simulink model "chydrbf_bruite_s"  (R2025a)
settings: Solver=ode45  StartTime=0.0  StopTime=50  MaxStep=1  MinStep=0.0001  RelTol=1e-8  AbsTol=1e-8  EnableMultiTasking=on
values from neighbouring files (symbols this model uses):
  F = [1 7.33333333333 21.7708333333 37 33.0208333333 11.4583333333]    [datahydr.mat]    (also in part4.m = ppfil(B,Aa,Tf); ppfil.m = real(poly(diag(r))))
  kw = 0.5    [datahydr.mat]    (also in initchydr.m)
  R = []    [bezout.m]    (also in datahydr.mat = [0 68.40625 346.729166667 625.944444444 808.75 137.5])
  S = []    [bezout.m]    (also in datahydr.mat = [1 9.5 38.1875 59.3541666667 159.118055556 0]; part4.m = [Sl 0])
  T = [12 88 261.25 444 396.25 137.5]    [datahydr.mat]    (also in part4.m = F*C(end)/B(end))
  Ta = 10    [datahydr.mat]    (also in initchydr.m)
  TI = 0.3    [datahydr.mat]    (also in initchydr.m)
  Tw = 1    [datahydr.mat]    (also in initchydr.m)
settings Model: Creator=pchevrel  LastModifiedBy=flo
settings SolverCC: AutoScaleAbsTol=off  AlgebraicLoopSolver=TrustRegion
settings DataIOCC: LimitDataPoints=on  SaveFormat=Array  SignalLoggingSaveFormat=ModelDataLogs  SaveOutput=off  SaveTime=off  ReturnWorkspaceOutputs=off  SignalLoggingName=sigsOut
settings OptimizationCC: ExpressionDepthLimit=2147483647.0  InitFltsAndDblsToZero=on  LifeSpan=inf
settings DebuggingCC: SaveWithParameterizedLinksMsg=none  UnderspecifiedInitializationDetection=Classic  MergeDetectMultiDrivingBlocksExec=none  SignalResolutionControl=TryResolveAllWithWarning  MultiTaskDSMMsg=warning  MultiTaskCondExecSysMsg=none  FcnCallInpInsideContextMsg=warning  UnconnectedInputMsg=warning  UnconnectedOutputMsg=warning  UnconnectedLineMsg=warning  StateNameClashWarn=warning  SFUnexpectedBacktrackingDiag=warning  SFNoUnconditionalDefaultTransitionDiag=warning  SFExecutionAtInitializationDiag=none  ArithmeticOperatorsInVariantConditions=warning
settings HardwareCC: ProdBitPerPointer=32.0  ProdBitPerSizeT=32.0  ProdBitPerPtrDiffT=32.0  ProdLargestAtomicFloat=None  ProdIntDivRoundTo=Undefined  ProdEndianess=Unspecified  ProdWordSize=32.0  ProdHWDeviceType=32-bit Generic  TargetUnknown=on
settings ModelReferenceCC: PropagateSignalLabelsOutOfModel=off
settings RTWCC: GPUComputeCapability=3.5
settings CodeAppCC: StateflowObjectComments=on
settings GRTTargetCC: TargetFcnLib=ansi_tfl_tmw.mat  TargetLangStandard=C89/C90 (ANSI)  CombineOutputUpdateFcns=off  GRTInterface=on
settings ConfigComp: CovMetricSettings=dw  CovSaveCumulativeToWorkspaceVar=on  CovSaveSingleToWorkspaceVar=on

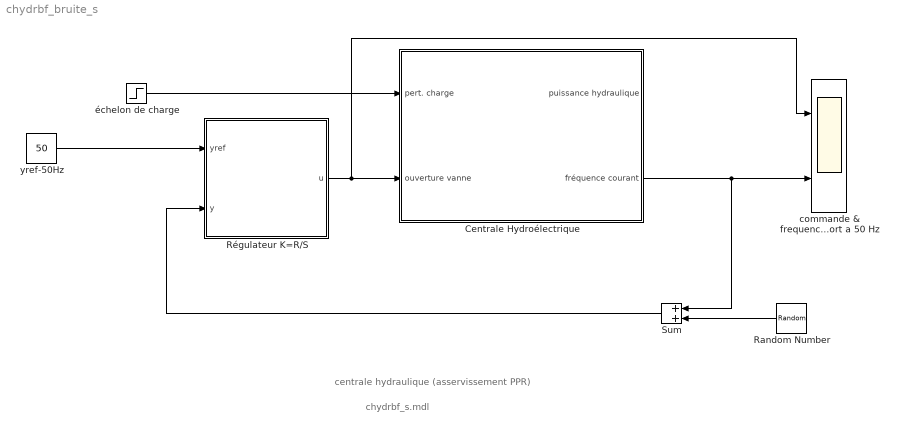
== system chydrbf_bruite_s ==
  note: chydrbf_s.mdl
  note: centrale hydraulique (asservissement PPR)
  Centrale Hydroélectrique : Subsystem
  Random Number : RandomNumber  Variance=5  SampleTime=0
  Régulateur K=R/S : Subsystem
  Sum : Sum  InputSameDT=on  SaturateOnIntegerOverflow=on  OutDataTypeStr=Inherit: Same as first input
  commande & frequence en relatif par rapport a 50 Hz : Scope  NumInputPorts=2
      settings: ActiveDisplayYMinimum=-113.05420502513749  ActiveDisplayYMaximum=679.22824500278932
  yref-50Hz : Constant  Value=50
  échelon de charge : Step  Time=20  After=10  SampleTime=0
  wires:
  Centrale Hydroélectrique/2(fréquence courant) -> commande & frequence en relatif par rapport a 50 Hz/2, Sum/1
  Régulateur K=R/S/1(u) -> Centrale Hydroélectrique/2(ouverture vanne), commande & frequence en relatif par rapport a 50 Hz/1
  yref-50Hz/1 -> Régulateur K=R/S/1(yref)
  échelon de charge/1 -> Centrale Hydroélectrique/1(pert. charge)
  Sum/1 -> Régulateur K=R/S/2(y)
  Random Number/1 -> Sum/2

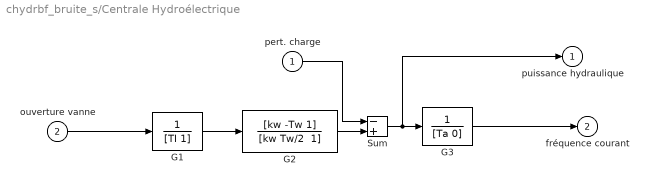
== system chydrbf_bruite_s/Centrale Hydroélectrique ==
  pert. charge : Inport
  ouverture vanne : Inport  Port=2
  G1 : TransferFcn  Denominator=[TI 1]
  G2 : TransferFcn  Numerator=[kw -Tw 1]  Denominator="[kw Tw/2  1]"
  G3 : TransferFcn  Denominator=[Ta 0]
  Sum : Sum  Inputs=-+  InputSameDT=on  SaturateOnIntegerOverflow=on  OutDataTypeStr=Inherit: Same as first input
  puissance hydraulique : Outport
  fréquence courant : Outport  Port=2
  wires:
  G2/1 -> Sum/2
  Sum/1 -> G3/1, puissance hydraulique/1
  G3/1 -> fréquence courant/1
  G1/1 -> G2/1
  pert. charge/1 -> Sum/1
  ouverture vanne/1 -> G1/1

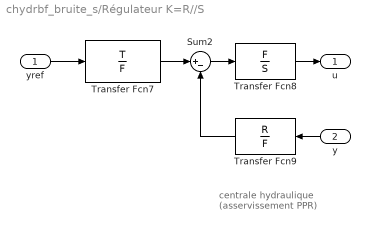
== system chydrbf_bruite_s/Régulateur K=R//S ==
  note: centrale hydraulique (asservissement PPR)
  yref : Inport
  y : Inport  Port=2
  Sum2 : Sum  Inputs=|+-  InputSameDT=on  SaturateOnIntegerOverflow=on  OutDataTypeStr=Inherit: Same as first input
  Transfer Fcn7 : TransferFcn  Numerator=T  Denominator=F
  Transfer Fcn8 : TransferFcn  Numerator=F  Denominator=S
  Transfer Fcn9 : TransferFcn  Numerator=R  Denominator=F
  u : Outport
  wires:
  Sum2/1 -> Transfer Fcn8/1
  Transfer Fcn7/1 -> Sum2/1
  Transfer Fcn9/1 -> Sum2/2
  yref/1 -> Transfer Fcn7/1
  Transfer Fcn8/1 -> u/1
  y/1 -> Transfer Fcn9/1
